simulink model "A4_PID_B_AttitudeDynamics"  (R2017b)
settings: Solver=VariableStepAuto  StartTime=0.0  StopTime=20  FixedStep=1  MaxStep=0.1  RelTol=1e-6  EnableMultiTasking=on
StopFcn:
  | attitudePlot = animateAttitude(rotmOut, 0.016);
  | attitudePlot.plotInit;
  | responsePlot(responseData, rotmOut, omegaRsOut, mechEnergyOut, mechPowerOut);
values from neighbouring files (symbols this model uses):
  J_sat = [2.5 2.5 2.5]    [AttitudeDynamicsData.m]
  PID_AA = struct(      'P', 2,          'I', 0.0002,     'D', 5           )    [AttitudeDynamicsData.m]
  PID_MPC = struct(      'P', 1.3,          'I', 0.0002,     'D', 3.02           )    [AttitudeDynamicsData.m]
  T_disturb = ones(1,3) * 0.1E-3    [AttitudeDynamicsData.m]
undefined symbols (not defined in the file or in its folder): DiscIntNeverNeededParam
libraries: SatelliteLibrary x16, simulink x1
(part 3 of 3)

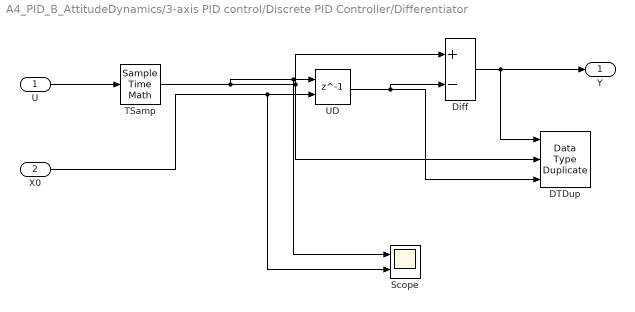
== system A4_PID_B_AttitudeDynamics/3-axis PID control/Discrete PID Controller/Differentiator ==
  U : Inport  SampleTime=SampleTime
  X0 : Inport  Port=2
  DTDup : DataTypeDuplicate  NumInputPorts=3
  Diff : Sum  Inputs=+-  OutMin=DifferentiatorOutMin  OutMax=DifferentiatorOutMax  OutDataTypeStr=Inherit: Inherit via back propagation  InputSameDT=on
  Scope : Scope  NumInputPorts=2
  TSamp : SampleTimeMath  TsampMathOp=/  TsampMathImp=Offline Scaling Adjustment
  UD : Delay  DelayLength=1  InitialConditionSource=Input port  InitialCondition=DifferentiatorICPrevScaledInput  InputProcessing=Inherited
      settings: InputPortMap=u0,p4
  Y : Outport  OutMin=DifferentiatorOutMin  OutMax=DifferentiatorOutMax  SampleTime=SampleTime
  wires:
  U/1 -> TSamp/1
  TSamp/1 -> Diff/1, DTDup/2, Scope/1, UD/1
  UD/1 -> Diff/2, DTDup/3
  Diff/1 -> Y/1, DTDup/1
  X0/1 -> Scope/2, UD/2

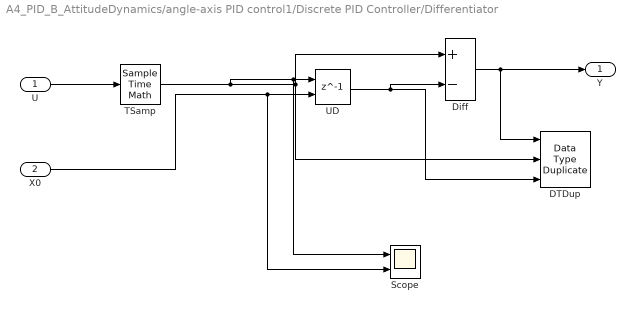
== system A4_PID_B_AttitudeDynamics/angle-axis PID control1/Discrete PID Controller/Differentiator ==
  U : Inport  SampleTime=SampleTime
  X0 : Inport  Port=2
  DTDup : DataTypeDuplicate  NumInputPorts=3
  Diff : Sum  Inputs=+-  OutMin=DifferentiatorOutMin  OutMax=DifferentiatorOutMax  OutDataTypeStr=Inherit: Inherit via back propagation  InputSameDT=on
  Scope : Scope  NumInputPorts=2
  TSamp : SampleTimeMath  TsampMathOp=/  TsampMathImp=Offline Scaling Adjustment
  UD : Delay  DelayLength=1  InitialConditionSource=Input port  InitialCondition=DifferentiatorICPrevScaledInput  InputProcessing=Inherited
      settings: InputPortMap=u0,p4
  Y : Outport  OutMin=DifferentiatorOutMin  OutMax=DifferentiatorOutMax  SampleTime=SampleTime
  wires:
  U/1 -> TSamp/1
  TSamp/1 -> Diff/1, DTDup/2, Scope/1, UD/1
  UD/1 -> Diff/2, DTDup/3
  Diff/1 -> Y/1, DTDup/1
  X0/1 -> Scope/2, UD/2

== matlab function A4_PID_B_AttitudeDynamics/Calculate Relative Attitude/minimum rotation quaternion ==
  data: q input; qPos output
function qPos = minRotation(q)
    % converts quaternion to form of smalest angle (last element always <0, 1] )
    if q(4) < 0
        qPos = -q;
    else
        qPos = q;
    end
end

== matlab function A4_PID_B_AttitudeDynamics/from SC to RS frame/sc frame to rs frame ==
  data: rotmSC input; Vrs output; rotmRS input; Vsc input
function ...
    Vrs               ...
  = sc2rs(            ...
    rotmSC,         ...
    rotmRS,         ...
    Vsc             ...
    )
    % transform vector in spacecraft (SC) frame into vector in
    % reactionsphere (RS) frame.
    Vrs = rotmRS' * rotmSC * Vsc;

end

== matlab function A4_PID_B_AttitudeDynamics/Calculate Relative Attitude/relative rotation matrix ==
  data: CAbs input; COrb input; CRel output
function CRel = rotmatRelative(...
    CAbs, ... absolute rotation matrix orientation (in inertial reference frame)
    COrb  ... orbital frame rotation matrix orientation
    )

CRel = COrb' * CAbs;
end

== matlab function A4_PID_B_AttitudeDynamics/Axis Angle Error/minimum rotation quaternion ==
  data: q input; qPos output
function qPos = minRotation(q)
    % converts quaternion to form of smalest angle (last element always <0, 1] )
    if q(4) < 0
        qPos = -q;
    else
        qPos = q;
    end
end

== matlab function A4_PID_B_AttitudeDynamics/Calculate Relative Attitude/relative quaternion ==
  data: qA input; qO input; qRel output
function qRel = quatRelative(...
    qA, ... absolute quaternion orientation (in inertial reference frame)
    qO  ... orbital frame quaternion orientation
    )
% Calculate the error quaternion
% q_... are standard quaternions with the vector part at the start

qOinv = [-qO(1:3); qO(4)];
qAmatrix = [ qA(4)  qA(3) -qA(2)  qA(1);...
            -qA(3)  qA(4)  qA(1)  qA(2);...
             qA(2) -qA(1)  qA(4)  qA(3);...
            -qA(1) -qA(2) -qA(3)  qA(4)];
qRel = qAmatrix * qOinv;
end

== matlab function A4_PID_B_AttitudeDynamics/from SC to RS frame1/sc frame to rs frame ==
  data: rotmSC input; Vrs output; rotmRS input; Vsc input
function ...
    Vrs               ...
  = sc2rs(            ...
    rotmSC,         ...
    rotmRS,         ...
    Vsc             ...
    )
    % transform vector in spacecraft (SC) frame into vector in
    % reactionsphere (RS) frame.
    Vrs = rotmRS' * rotmSC * Vsc;

end
